simulink model "Washing_machine"  (R2024b)
settings: Solver=VariableStepAuto  StartTime=0.0  StopTime=inf  RelTol=1e-3
settings Model: Creator=ksamb  LastModifiedBy=ksamb

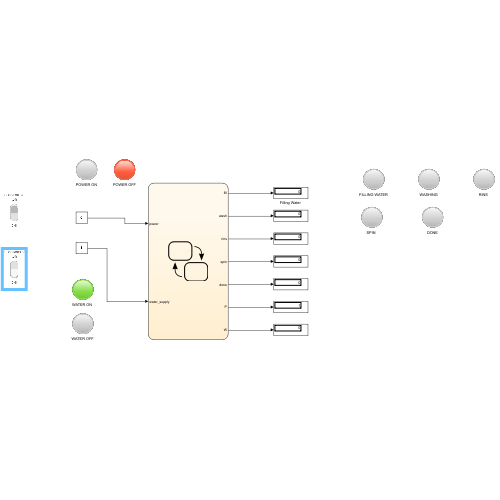
[thumbnail: Simulink's stored preview of the top-level diagram]
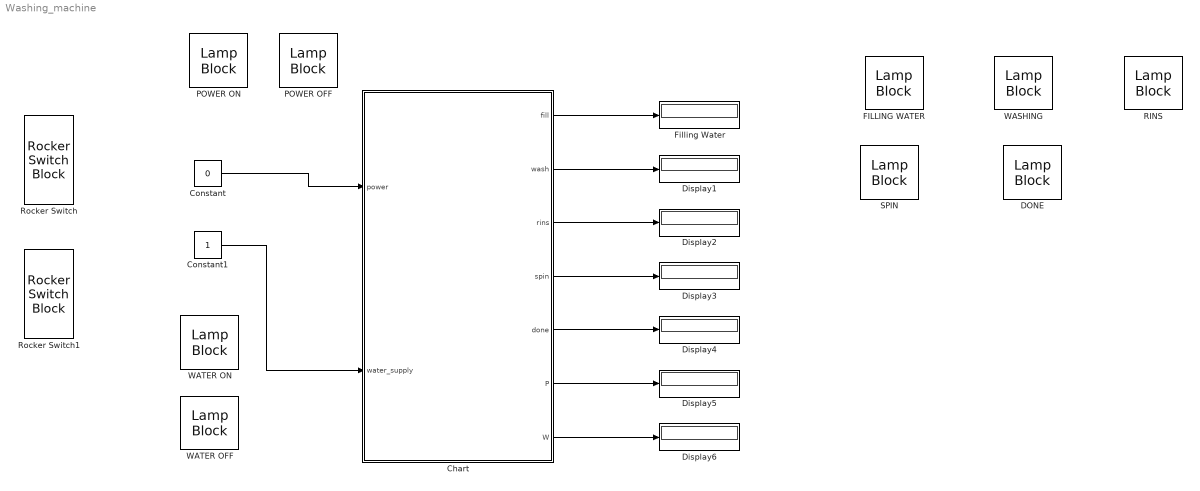
== system Washing_machine ==
  Chart : Stateflow chart  TreatAsAtomicUnit=on
  Constant : Constant  Value=0
  Constant1 : Constant
  DONE : LampBlock  LabelPosition=Hide
  Display{1..6} (6 alike) : Display
  FILLING WATER : LampBlock  LabelPosition=Hide
  "Filling Water " : Display
  POWER OFF : LampBlock  LabelPosition=Hide
  POWER ON : LampBlock  LabelPosition=Hide
  "RINS " : LampBlock  LabelPosition=Hide
  Rocker Switch : RockerSwitchBlock
      settings: Values={{'Off', 'On'}, [0 1]}
  Rocker Switch1 : RockerSwitchBlock
      settings: Values={{'Off', 'On'}, [0 1]}
  "SPIN " : LampBlock  LabelPosition=Hide
  WASHING : LampBlock  LabelPosition=Hide
  WATER OFF : LampBlock  LabelPosition=Hide
  "WATER ON " : LampBlock  LabelPosition=Hide
  wires:
  Constant/1 -> Chart/1(power)
  Constant1/1 -> Chart/2(water_supply)
  Chart/1(fill) -> "Filling Water "/1
  Chart/2(wash) -> Display1/1
  Chart/3(rins) -> Display2/1
  Chart/4(spin) -> Display3/1
  Chart/5(done) -> Display4/1
  Chart/6(P) -> Display5/1
  Chart/7(W) -> Display6/1

== stateflow chart Washing_machine/Chart ==
  state power_on
  state water
    W=0;
  state FILL
    entry:fill =1;
  state WASH
    entry:
    fill=0,wash=1;
  state RINS
    entry:
    wash=0,rins=1;
  state SPIN
    entry:
    rins=0,spin=1;
  state DONE
    entry:
    spin=0,done=1;
  state water_suppl_ind
    during:
    if water_supply==0
    W=1;
    else
    W=0;
    end
  state power_Indicator
    during:
    if power==0
    P=1;
    W=0;
    fill=0;
    wash=0;
    rins=0;
    spin=0;
    else
    P=0;
    end
  (default) -> power_on : {power == 1}
  water -> FILL [order 1] : [water_supply == 1 &&...
      | power == 1]
  FILL -> WASH [order 1] : after(5,sec)
      | [power == 1]
  WASH -> RINS [order 1] : after(5,sec)
  RINS -> SPIN [order 1] : after(5,sec)
  SPIN -> DONE [order 1] : after(5,sec)
  power_on -> water [order 1] : [power == 1]...
      | {after(3,sec)}
  power_Indicator -> power_on : [power == 1]
  power_on -> power_Indicator [order 2] : [power == 0]
  water_suppl_ind -> water : [water_supply ==1]
  water -> water_suppl_ind [order 2] : [water_supply ==0]
  FILL -> (junction 40) [order 2] : [power == 0]
  DONE -> (junction 40) : [power == 0]
  SPIN -> (junction 40) [order 2] : [power == 0]
  WASH -> (junction 40) [order 2] : [power == 0]
  RINS -> (junction 40) [order 2] : [power == 0]
  (junction 40) -> power_Indicator : [power == 0]
  data: fill output; wash output; rins output; spin output; done output; power input; water_supply input; P output; W output
